simulink model "problem5"  (R2019a)
settings: Solver=VariableStepAuto  StartTime=0.0  StopTime=10000  RelTol=1e-3
undefined symbols (not defined in the file): m, n
settings Model: Creator=Avery Peiffer  LastModifiedBy=Avery Peiffer

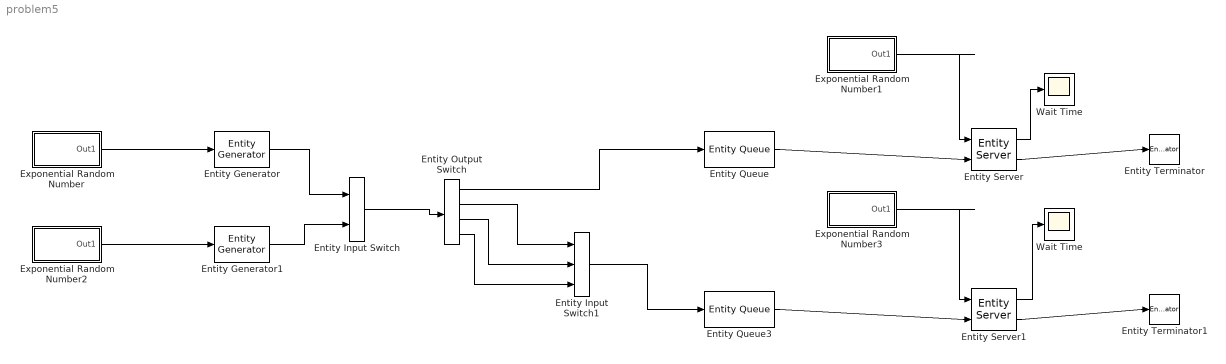
== system problem5 ==
  Entity Input Switch : EntityInputSwitch  InputPortMessageModes=m,m  OutputPortMessageModes=m
  Entity Input Switch1 : EntityInputSwitch  InputPortMessageModes=m,m,m  OutputPortMessageModes=m  NumberInputPorts=3
      settings: InputPortMap=u1,u2,u3
  Entity Output Switch : EntityOutputSwitch  InputPortMessageModes=m  OutputPortMessageModes=m,m,m,m  NumberOutputPorts=4  SwitchingCriterion=Equiprobable  Seed=4  SwitchAttributeName=Attribute1
      settings: OutputPortMap=o0,o1,o2,o3
  Entity Generator : EntityGenerator  OutputPortMessageModes=m  TimeSource=Signal port  EntityType=Structured  EntityTypeName=Entity
      settings: InputPortMap=u1
  Entity Generator1 : EntityGenerator  OutputPortMessageModes=m  TimeSource=Signal port  EntityType=Structured  EntityTypeName=Entity
      settings: InputPortMap=u1
  Entity Queue : EntityQueue  InputPortMessageModes=m  OutputPortMessageModes=m  Capacity=1
      settings: OutputPortMap=o5
  Entity Queue3 : EntityQueue  InputPortMessageModes=m  OutputPortMessageModes=m  Capacity=1
      settings: OutputPortMap=o5
  Entity Server : EntityServer  InputPortMessageModes=n,m  OutputPortMessageModes=n,m  Capacity=1  ServiceTimeSource=Signal port  AverageWait=on
      settings: InputPortMap=u0,u2  OutputPortMap=o4,o9
  Entity Server1 : EntityServer  InputPortMessageModes=n,m  OutputPortMessageModes=n,m  Capacity=1  ServiceTimeSource=Signal port  AverageWait=on
      settings: InputPortMap=u0,u2  OutputPortMap=o4,o9
  Entity Terminator : EntityTerminator  InputPortMessageModes=m
  Entity Terminator1 : EntityTerminator  InputPortMessageModes=m
  Exponential Random Number : Subsystem  mask(Exponential Random Number){mean=.111, seed=16}
      mask prompts: seed "Random Seed"
      mask help: This block generate a random number with exponential distribution.
      mask Display: disp(['mean=' num2str(mean,2)],"texmode","on");
  Exponential Random Number1 : Subsystem  mask(Exponential Random Number){mean=.0714, seed=24}
      mask prompts: seed "Random Seed"
      mask help: This block generate a random number with exponential distribution.
      mask Display: disp(['mean=' num2str(mean,2)],"texmode","on");
  Exponential Random Number2 : Subsystem  mask(Exponential Random Number){mean=.333, seed=24}
      mask prompts: seed "Random Seed"
      mask help: This block generate a random number with exponential distribution.
      mask Display: disp(['mean=' num2str(mean,2)],"texmode","on");
  Exponential Random Number3 : Subsystem  mask(Exponential Random Number){mean=.0825, seed=28}
      mask prompts: seed "Random Seed"
      mask help: This block generate a random number with exponential distribution.
      mask Display: disp(['mean=' num2str(mean,2)],"texmode","on");
  Wait Time : Scope
  "Wait Time " : Scope
  wires:
  Exponential Random Number/1(Out1) -> Entity Generator/1
  Exponential Random Number2/1(Out1) -> Entity Generator1/1
  Entity Server1/2 -> Entity Terminator1/1
  Exponential Random Number3/1(Out1) -> Entity Server1/1
  Exponential Random Number1/1(Out1) -> Entity Server/1
  Entity Queue/1 -> Entity Server/2
  Entity Server/2 -> Entity Terminator/1
  Entity Server/1 -> Wait Time/1
  Entity Server1/1 -> "Wait Time "/1
  Entity Input Switch/1 -> Entity Output Switch/1
  Entity Generator1/1 -> Entity Input Switch/2
  Entity Generator/1 -> Entity Input Switch/1
  Entity Output Switch/1 -> Entity Queue/1
  Entity Queue3/1 -> Entity Server1/2
  Entity Output Switch/2 -> Entity Input Switch1/1
  Entity Output Switch/3 -> Entity Input Switch1/2
  Entity Output Switch/4 -> Entity Input Switch1/3
  Entity Input Switch1/1 -> Entity Queue3/1

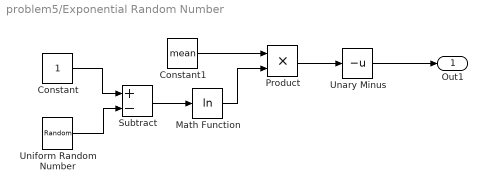
== system problem5/Exponential Random Number ==
  Constant : Constant
  Constant1 : Constant  Value=mean
  Math Function : Math  Operator=log  SaturateOnIntegerOverflow=on
  Product : Product  RndMeth=Zero
  Subtract : Sum  Inputs=+-
  Unary Minus : UnaryMinus
  Uniform Random Number : UniformRandomNumber  Minimum=0  Seed=seed
  Out1 : Outport  VectorParamsAs1DForOutWhenUnconnected=on
  wires:
  Subtract/1 -> Math Function/1
  Math Function/1 -> Product/2
  Unary Minus/1 -> Out1/1
  Product/1 -> Unary Minus/1
  Constant/1 -> Subtract/1
  Uniform Random Number/1 -> Subtract/2
  Constant1/1 -> Product/1

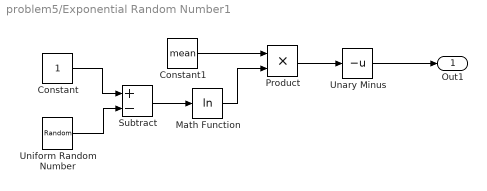
== system problem5/Exponential Random Number1 ==
  Constant : Constant
  Constant1 : Constant  Value=mean
  Math Function : Math  Operator=log  SaturateOnIntegerOverflow=on
  Product : Product  RndMeth=Zero
  Subtract : Sum  Inputs=+-
  Unary Minus : UnaryMinus
  Uniform Random Number : UniformRandomNumber  Minimum=0  Seed=seed
  Out1 : Outport  VectorParamsAs1DForOutWhenUnconnected=on
  wires:
  Subtract/1 -> Math Function/1
  Math Function/1 -> Product/2
  Unary Minus/1 -> Out1/1
  Product/1 -> Unary Minus/1
  Constant/1 -> Subtract/1
  Uniform Random Number/1 -> Subtract/2
  Constant1/1 -> Product/1

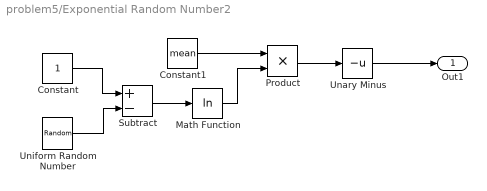
== system problem5/Exponential Random Number2 ==
  Constant : Constant
  Constant1 : Constant  Value=mean
  Math Function : Math  Operator=log  SaturateOnIntegerOverflow=on
  Product : Product  RndMeth=Zero
  Subtract : Sum  Inputs=+-
  Unary Minus : UnaryMinus
  Uniform Random Number : UniformRandomNumber  Minimum=0  Seed=seed
  Out1 : Outport  VectorParamsAs1DForOutWhenUnconnected=on
  wires:
  Subtract/1 -> Math Function/1
  Math Function/1 -> Product/2
  Unary Minus/1 -> Out1/1
  Product/1 -> Unary Minus/1
  Constant/1 -> Subtract/1
  Uniform Random Number/1 -> Subtract/2
  Constant1/1 -> Product/1

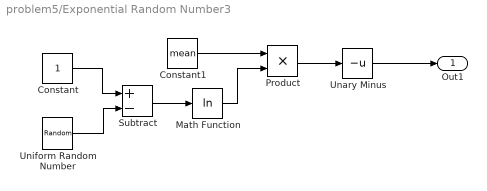
== system problem5/Exponential Random Number3 ==
  Constant : Constant
  Constant1 : Constant  Value=mean
  Math Function : Math  Operator=log  SaturateOnIntegerOverflow=on
  Product : Product  RndMeth=Zero
  Subtract : Sum  Inputs=+-
  Unary Minus : UnaryMinus
  Uniform Random Number : UniformRandomNumber  Minimum=0  Seed=seed
  Out1 : Outport  VectorParamsAs1DForOutWhenUnconnected=on
  wires:
  Subtract/1 -> Math Function/1
  Math Function/1 -> Product/2
  Unary Minus/1 -> Out1/1
  Product/1 -> Unary Minus/1
  Constant/1 -> Subtract/1
  Uniform Random Number/1 -> Subtract/2
  Constant1/1 -> Product/1
